simulink model "DoubleInvertedPendulum"  (R2015a)
settings: Solver=ode45  StartTime=0.0  StopTime=20  RelTol=1e-3
values from neighbouring files (symbols this model uses):
  A = [ ... (first row only)    [DoubleInvertedPendulum_config.m]
  B = [ ... (first row only)    [DoubleInvertedPendulum_config.m]
  g = 9.8    [DoubleInvertedPendulum_config.m]
  gain = lqr( A ,B, Q, R )    [DoubleInvertedPendulum_config.m]
  J1 = 1.0    (= 1)    [DoubleInvertedPendulum_config.m]
  J2 = 1.0    (= 1)    [DoubleInvertedPendulum_config.m]
  l1 = 2.0    (= 2)    [DoubleInvertedPendulum_config.m]
  l2 = 1.0    (= 1)    [DoubleInvertedPendulum_config.m]
  lg1 = 1.2    [DoubleInvertedPendulum_config.m]
  lg2 = 0.5    [DoubleInvertedPendulum_config.m]
  m0 = 5.0    (= 5)    [DoubleInvertedPendulum_config.m]
  m1 = 1.0    (= 1)    [DoubleInvertedPendulum_config.m]
  m2 = 1.0    (= 1)    [DoubleInvertedPendulum_config.m]
settings Model: Creator=hamada  LastModifiedBy=hamada

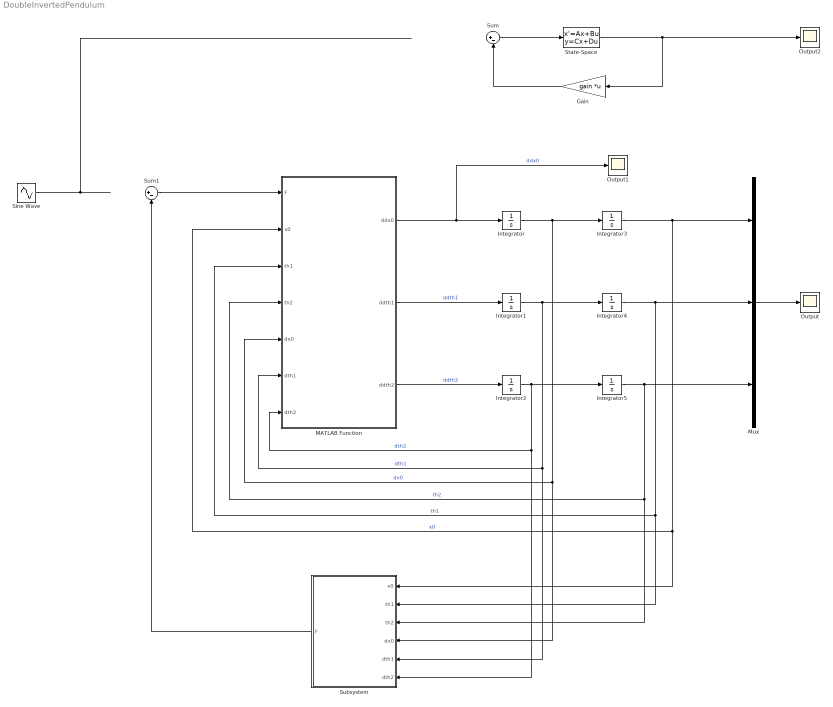
== system DoubleInvertedPendulum ==
  Gain : Gain  Gain=gain  Multiplication=Matrix(K*u)
  Integrator{,1..3} (4 alike) : Integrator
  Integrator4 : Integrator  InitialCondition=5*pi/180
  Integrator5 : Integrator  InitialCondition=5*pi/180
  MATLAB Function : MATLAB Function  TreatAsAtomicUnit=on
  Mux : Mux  Inputs=3
  Output : Scope
      settings: SaveName=Output  SampleInput=on  SampleTime=0.1
  Output1 : Scope
      settings: SaveName=Output1  SampleInput=on  SampleTime=0.1
  Output2 : Scope
      settings: SaveName=Output2  SampleInput=on  SampleTime=0.1
  Sine Wave : Sin  Amplitude=10  Frequency=1*2*pi  SampleTime=0
  State-Space : StateSpace  A=A  B=B  C=eye(6)  D=zeros(6,1)  X0=[0;5*pi/180;0;0;0;0]
  Subsystem : Subsystem
  Sum : Sum  Inputs=|+-
  Sum1 : Sum  Inputs=|+-
  wires:
  MATLAB Function/1(ddx0) -> Output1/1, Integrator/1  "ddx0"
  MATLAB Function/2(ddth1) -> Integrator1/1  "ddth1"
  MATLAB Function/3(ddth2) -> Integrator2/1  "ddth2"
  Integrator/1 -> Subsystem/4(dx0), MATLAB Function/5(dx0), Integrator3/1  "dx0"
  Integrator1/1 -> Subsystem/5(dth1), MATLAB Function/6(dth1), Integrator4/1  "dth1"
  Integrator2/1 -> Subsystem/6(dth2), MATLAB Function/7(dth2), Integrator5/1  "dth2"
  Integrator3/1 -> Mux/1, MATLAB Function/2(x0), Subsystem/1(x0)  "x0"
  Integrator4/1 -> Mux/2, Subsystem/2(th1), MATLAB Function/3(th1)  "th1"
  Integrator5/1 -> Subsystem/3(th2), MATLAB Function/4(th2), Mux/3  "th2"
  Sine Wave/1 -> ?
  Mux/1 -> Output/1
  State-Space/1 -> Output2/1, Gain/1
  Sum/1 -> State-Space/1
  Gain/1 -> Sum/2
  Sum1/1 -> MATLAB Function/1(F)
  Subsystem/1(F) -> Sum1/2

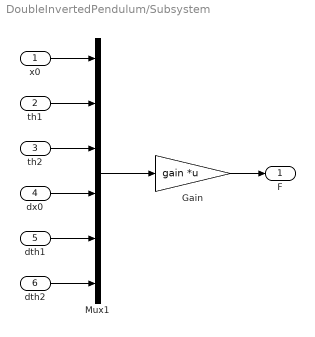
== system DoubleInvertedPendulum/Subsystem ==
  x0 : Inport
  th1 : Inport  Port=2
  th2 : Inport  Port=3
  dx0 : Inport  Port=4
  dth1 : Inport  Port=5
  dth2 : Inport  Port=6
  Gain : Gain  Gain=gain  Multiplication=Matrix(K*u)
  Mux1 : Mux  Inputs=6
  F : Outport
  wires:
  Mux1/1 -> Gain/1
  dth2/1 -> Mux1/6
  dx0/1 -> Mux1/4
  th1/1 -> Mux1/2
  dth1/1 -> Mux1/5
  x0/1 -> Mux1/1
  th2/1 -> Mux1/3
  Gain/1 -> F/1

== matlab function DoubleInvertedPendulum/MATLAB Function ==
  data: F input double size=1; x0 input double size=1; ddx0 output double size=1; ddth1 output double size=1; ddth2 output double size=1; th1 input double size=1; th2 input double size=1; dx0 input double size=1; dth1 input double size=1; dth2 input double size=1; lg1 parameter double size=1; l1 parameter double size=1; lg2 parameter double size=1; l2 parameter double size=1; m0 parameter double size=1; m1 parameter double size=1; m2 parameter double size=1; J1 parameter double size=1; J2 parameter double size=1; g parameter double size=1
function [ ddx0, ddth1, ddth2 ] = fcn( F, x0, th1, th2, dx0, dth1, dth2, lg1, l1, lg2, l2, m0, m1, m2, J1, J2, g )
    %#codegen
    ddx0 = (((g*l1^2*lg2^2*m2^3+(g*lg1^2*lg2^2*m1+J1*g*lg2^2)*m2^2)*cos(th2+th1)+(l1^2*lg2^3*m2^3*(cos(th2)^2-1)+(-lg1^2*lg2^3*m1-J1*lg2^3-J2*l1^2*lg2)*m2^2+(-J2*lg1^2*lg2*m1-J1*J2*lg2)*m2)*(dth2)^2+(dth1)*(l1^2*lg2^3*m2^3*(2*cos(th2)^2-2)+(-2*lg1^2*lg2^3*m1-2*J1*lg2^3-2*J2*l1^2*lg2)*m2^2+(-2*J2*lg1^2*lg2*m1-2*J1*J2*lg2)*m2)*(dth2)+(dth1)^2*(l1^2*lg2^3*m2^3*(cos(th2)^2-1)+(-lg1^2*lg2^3*m1-J1*lg2^3-J2*l1^2*lg2)*m2^2+(-J2*lg1^2*lg2*m1-J1*J2*lg2)*m2)+cos(th1)*(-g*l1^2*lg2^2*m2^3*cos(th2)-g*l1*lg1*lg2^2*m1*m2^2*cos(th2)))*sin(th2+th1)+(-l1^2*lg2^3*m2^3*cos(th2)*sin(th2)*(dth2)^2-2*l1^2*lg2^3*m2^3*(dth1)*cos(th2)*sin(th2)*(dth2)+(dth1)^2*(m2^3*(-l1^2*lg2^3*cos(th2)*sin(th2)-l1^3*lg2^2*sin(th2))+m2^2*(-l1*lg1^2*lg2^2*m1*sin(th2)-J1*l1*lg2^2*sin(th2)))+sin(th1)*(-g*l1^2*lg2^2*m2^3*cos(th2)-g*l1*lg1*lg2^2*m1*m2^2*cos(th2)))*cos(th2+th1)+cos(th1)*(m2^2*(l1*lg1*lg2^3*m1*sin(th2)+J2*l1^2*lg2*sin(th2))+l1^2*lg2^3*m2^3*sin(th2)+J2*l1*lg1*lg2*m1*m2*sin(th2))*(dth2)^2+cos(th1)*(dth1)*(m2^2*(2*l1*lg1*lg2^3*m1*sin(th2)+2*J2*l1^2*lg2*sin(th2))+2*l1^2*lg2^3*m2^3*sin(th2)+2*J2*l1*lg1*lg2*m1*m2*sin(th2))*(dth2)+(dth1)^2*(cos(th1)*(m2^2*(m1*(l1^2*lg1*lg2^2*cos(th2)*sin(th2)+l1*lg1*lg2^3*sin(th2))+J2*l1^2*lg2*sin(th2))+m2^3*(l1^3*lg2^2*cos(th2)*sin(th2)+l1^2*lg2^3*sin(th2))+J2*l1*lg1*lg2*m1*m2*sin(th2))+sin(th1)*(l1^3*lg2^2*m2^3*(cos(th2)^2-1)+m2^2*(lg2^2*m1*(l1^2*lg1*(cos(th2)^2-1)-l1*lg1^2)-J1*l1*lg2^2-J2*l1^3)+(-lg1^3*lg2^2*m1^2+(-J1*lg1*lg2^2-J2*l1*lg1^2-J2*l1^2*lg1)*m1-J1*J2*l1)*m2-J2*lg1^3*m1^2-J1*J2*lg1*m1))+F*l1^2*lg2^2*m2^2*(cos(th2)^2-1)+(g*l1^2*lg2^2*m2^3+(2*g*l1*lg1*lg2^2*m1+J2*g*l1^2)*m2^2+(g*lg1^2*lg2^2*m1^2+2*J2*g*l1*lg1*m1)*m2+J2*g*lg1^2*m1^2)*cos(th1)*sin(th1)+(-F*lg1^2*lg2^2*m1-F*J1*lg2^2-F*J2*l1^2)*m2-F*J2*lg1^2*m1-F*J1*J2)/((l1^2*lg2^2*m2^3+(lg1^2*lg2^2*m1+J1*lg2^2)*m2^2)*cos(th2+th1)^2+cos(th1)*(-2*l1^2*lg2^2*m2^3*cos(th2)-2*l1*lg1*lg2^2*m1*m2^2*cos(th2))*cos(th2+th1)+l1^2*lg2^2*m2^3*(cos(th2)^2-1)+m2^2*(l1^2*lg2^2*m0*(cos(th2)^2-1)+lg2^2*m1*(l1^2*(cos(th2)^2-1)-lg1^2)-J1*lg2^2-J2*l1^2)+(l1^2*lg2^2*m2^3+(2*l1*lg1*lg2^2*m1+J2*l1^2)*m2^2+(lg1^2*lg2^2*m1^2+2*J2*l1*lg1*m1)*m2+J2*lg1^2*m1^2)*cos(th1)^2+(-lg1^2*lg2^2*m1^2+(-lg1^2*lg2^2*m0-J1*lg2^2-J2*lg1^2-J2*l1^2)*m1+(-J1*lg2^2-J2*l1^2)*m0-J1*J2)*m2-J2*lg1^2*m1^2+(-J2*lg1^2*m0-J1*J2)*m1-J1*J2*m0);
    ddth1 = -(((l1*lg2^3*m2^3*cos(th2)*(dth2)^2+2*l1*lg2^3*m2^3*(dth1)*cos(th2)*(dth2)+l1*lg2^3*m2^3*(dth1)^2*cos(th2)+(g*l1*lg2^2*m2^3+g*lg1*lg2^2*m1*m2^2)*cos(th1))*cos(th2+th1)+(-l1*lg2^3*m2^3+(-lg1*lg2^3*m1-J2*l1*lg2)*m2^2-J2*lg1*lg2*m1*m2)*cos(th1)*(dth2)^2+(-2*l1*lg2^3*m2^3+(-2*lg1*lg2^3*m1-2*J2*l1*lg2)*m2^2-2*J2*lg1*lg2*m1*m2)*cos(th1)*(dth1)*(dth2)+m2^2*(-g*l1*lg2^2*m1*cos(th2)-g*l1*lg2^2*m0*cos(th2))-g*l1*lg2^2*m2^3*cos(th2)+(-l1*lg2^3*m2^3+(-lg1*lg2^3*m1-J2*l1*lg2)*m2^2-J2*lg1*lg2*m1*m2)*cos(th1)*(dth1)^2)*sin(th2+th1)+(-l1*lg2^3*m2^3*sin(th2)*(dth2)^2-2*l1*lg2^3*m2^3*(dth1)*sin(th2)*(dth2)-l1*lg2^3*m2^3*(dth1)^2*sin(th2)+(-g*l1*lg2^2*m2^3-g*lg1*lg2^2*m1*m2^2)*sin(th1))*cos(th2+th1)^2+((dth1)^2*(cos(th1)*(-l1^2*lg2^2*m2^3*sin(th2)-l1*lg1*lg2^2*m1*m2^2*sin(th2))+sin(th1)*(l1^2*lg2^2*m2^3*cos(th2)+l1*lg1*lg2^2*m1*m2^2*cos(th2)))+F*l1*lg2^2*m2^2*cos(th2))*cos(th2+th1)+(m2^2*(l1*lg2^3*m1*sin(th2)+l1*lg2^3*m0*sin(th2)+J2*l1*lg2*sin(th2))+m2*(J2*l1*lg2*m1*sin(th2)+J2*l1*lg2*m0*sin(th2))+l1*lg2^3*m2^3*sin(th2))*(dth2)^2+(dth1)*(m2^2*(2*l1*lg2^3*m1*sin(th2)+2*l1*lg2^3*m0*sin(th2)+2*J2*l1*lg2*sin(th2))+m2*(2*J2*l1*lg2*m1*sin(th2)+2*J2*l1*lg2*m0*sin(th2))+2*l1*lg2^3*m2^3*sin(th2))*(dth2)+(dth1)^2*(m2^2*(m1*(l1^2*lg2^2*cos(th2)*sin(th2)+l1*lg2^3*sin(th2))+m0*(l1^2*lg2^2*cos(th2)*sin(th2)+l1*lg2^3*sin(th2))+J2*l1*lg2*sin(th2))+m2^3*(l1^2*lg2^2*cos(th2)*sin(th2)+l1*lg2^3*sin(th2))+m2*(J2*l1*lg2*m1*sin(th2)+J2*l1*lg2*m0*sin(th2))+(-l1^2*lg2^2*m2^3+(-2*l1*lg1*lg2^2*m1-J2*l1^2)*m2^2+(-lg1^2*lg2^2*m1^2-2*J2*l1*lg1*m1)*m2-J2*lg1^2*m1^2)*cos(th1)*sin(th1))+(g*l1*lg2^2*m2^3+((g*lg1+g*l1)*lg2^2*m1+g*l1*lg2^2*m0+J2*g*l1)*m2^2+(g*lg1*lg2^2*m1^2+(g*lg1*lg2^2*m0+J2*g*lg1+J2*g*l1)*m1+J2*g*l1*m0)*m2+J2*g*lg1*m1^2+J2*g*lg1*m0*m1)*sin(th1)+(-F*l1*lg2^2*m2^2+(-F*lg1*lg2^2*m1-F*J2*l1)*m2-F*J2*lg1*m1)*cos(th1))/((l1^2*lg2^2*m2^3+(lg1^2*lg2^2*m1+J1*lg2^2)*m2^2)*cos(th2+th1)^2+cos(th1)*(-2*l1^2*lg2^2*m2^3*cos(th2)-2*l1*lg1*lg2^2*m1*m2^2*cos(th2))*cos(th2+th1)+l1^2*lg2^2*m2^3*(cos(th2)^2-1)+m2^2*(l1^2*lg2^2*m0*(cos(th2)^2-1)+lg2^2*m1*(l1^2*(cos(th2)^2-1)-lg1^2)-J1*lg2^2-J2*l1^2)+(l1^2*lg2^2*m2^3+(2*l1*lg1*lg2^2*m1+J2*l1^2)*m2^2+(lg1^2*lg2^2*m1^2+2*J2*l1*lg1*m1)*m2+J2*lg1^2*m1^2)*cos(th1)^2+(-lg1^2*lg2^2*m1^2+(-lg1^2*lg2^2*m0-J1*lg2^2-J2*lg1^2-J2*l1^2)*m1+(-J1*lg2^2-J2*l1^2)*m0-J1*J2)*m2-J2*lg1^2*m1^2+(-J2*lg1^2*m0-J1*J2)*m1-J1*J2*m0);
    ddth2 = ((((m2^3*(l1*lg2^3*cos(th2)+l1^2*lg2^2)+(lg1^2*lg2^2*m1+J1*lg2^2)*m2^2)*(dth2)^2+(dth1)*(m2^3*(2*l1*lg2^3*cos(th2)+2*l1^2*lg2^2)+(2*lg1^2*lg2^2*m1+2*J1*lg2^2)*m2^2)*(dth2)+(dth1)^2*(m2^3*(l1*lg2^3*cos(th2)+l1^2*lg2^2)+(lg1^2*lg2^2*m1+J1*lg2^2)*m2^2)+(g*l1*lg2^2*m2^3+g*lg1*lg2^2*m1*m2^2)*cos(th1))*cos(th2+th1)+cos(th1)*(m2^2*(m1*(-l1*lg1*lg2^2*cos(th2)-lg1*lg2^3)-J2*l1*lg2)+m2^3*(-l1^2*lg2^2*cos(th2)-l1*lg2^3)-J2*lg1*lg2*m1*m2)*(dth2)^2+cos(th1)*(dth1)*(m2^2*(m1*(-2*l1*lg1*lg2^2*cos(th2)-2*lg1*lg2^3)-2*J2*l1*lg2)+m2^3*(-2*l1^2*lg2^2*cos(th2)-2*l1*lg2^3)-2*J2*lg1*lg2*m1*m2)*(dth2)+cos(th1)*(dth1)^2*(m2^2*(m1*(-l1*lg1*lg2^2*cos(th2)-lg1*lg2^3)-J2*l1*lg2)+m2^3*(-l1^2*lg2^2*cos(th2)-l1*lg2^3)-J2*lg1*lg2*m1*m2)+m2^2*(m1*((-g*lg1^2-g*l1^2)*lg2-g*l1*lg2^2*cos(th2))+m0*(-g*l1*lg2^2*cos(th2)-g*l1^2*lg2)-J1*g*lg2)+m2^3*(-g*l1*lg2^2*cos(th2)-g*l1^2*lg2)+(g*l1^2*lg2*m2^3+2*g*l1*lg1*lg2*m1*m2^2+g*lg1^2*lg2*m1^2*m2)*cos(th1)^2+(-g*lg1^2*lg2*m1^2+(-g*lg1^2*lg2*m0-J1*g*lg2)*m1-J1*g*lg2*m0)*m2)*sin(th2+th1)+(-l1*lg2^3*m2^3*sin(th2)*(dth2)^2-2*l1*lg2^3*m2^3*(dth1)*sin(th2)*(dth2)-l1*lg2^3*m2^3*(dth1)^2*sin(th2)+(-g*l1*lg2^2*m2^3-g*lg1*lg2^2*m1*m2^2)*sin(th1))*cos(th2+th1)^2+(cos(th1)*(-l1^2*lg2^2*m2^3*sin(th2)-l1*lg1*lg2^2*m1*m2^2*sin(th2))*(dth2)^2+cos(th1)*(dth1)*(-2*l1^2*lg2^2*m2^3*sin(th2)-2*l1*lg1*lg2^2*m1*m2^2*sin(th2))*(dth2)+(dth1)^2*(cos(th1)*(-2*l1^2*lg2^2*m2^3*sin(th2)-2*l1*lg1*lg2^2*m1*m2^2*sin(th2))+sin(th1)*(m2^2*(m1*(l1*lg1*lg2^2*cos(th2)+(l1*lg1^2+l1^2*lg1)*lg2)+J1*l1*lg2)+m2^3*(l1^2*lg2^2*cos(th2)+l1^3*lg2)+(lg1^3*lg2*m1^2+J1*lg1*lg2*m1)*m2))+m2^2*(F*l1*lg2^2*cos(th2)+F*l1^2*lg2)+(-g*l1^2*lg2*m2^3-2*g*l1*lg1*lg2*m1*m2^2-g*lg1^2*lg2*m1^2*m2)*cos(th1)*sin(th1)+(F*lg1^2*lg2*m1+F*J1*lg2)*m2)*cos(th2+th1)+(m2^2*(m1*(l1^2*lg2^2*cos(th2)*sin(th2)+l1*lg2^3*sin(th2))+m0*(l1^2*lg2^2*cos(th2)*sin(th2)+l1*lg2^3*sin(th2))+J2*l1*lg2*sin(th2))+m2^3*(l1^2*lg2^2*cos(th2)*sin(th2)+l1*lg2^3*sin(th2))+m2*(J2*l1*lg2*m1*sin(th2)+J2*l1*lg2*m0*sin(th2)))*(dth2)^2+(dth1)*(m2^2*(m1*(2*l1^2*lg2^2*cos(th2)*sin(th2)+2*l1*lg2^3*sin(th2))+m0*(2*l1^2*lg2^2*cos(th2)*sin(th2)+2*l1*lg2^3*sin(th2))+2*J2*l1*lg2*sin(th2))+m2^3*(2*l1^2*lg2^2*cos(th2)*sin(th2)+2*l1*lg2^3*sin(th2))+m2*(2*J2*l1*lg2*m1*sin(th2)+2*J2*l1*lg2*m0*sin(th2)))*(dth2)+(dth1)^2*(m2^2*(m1*(lg2*(l1*lg1^2*sin(th2)+l1^3*sin(th2))+2*l1^2*lg2^2*cos(th2)*sin(th2)+l1*lg2^3*sin(th2))+m0*(2*l1^2*lg2^2*cos(th2)*sin(th2)+l1*lg2^3*sin(th2)+l1^3*lg2*sin(th2))+(J2+J1)*l1*lg2*sin(th2))+m2*(m1*(l1*lg1^2*lg2*m0*sin(th2)+(J2+J1)*l1*lg2*sin(th2))+l1*lg1^2*lg2*m1^2*sin(th2)+(J2+J1)*l1*lg2*m0*sin(th2))+m2^3*(2*l1^2*lg2^2*cos(th2)*sin(th2)+l1*lg2^3*sin(th2)+l1^3*lg2*sin(th2))+cos(th1)^2*(-l1^3*lg2*m2^3*sin(th2)-2*l1^2*lg1*lg2*m1*m2^2*sin(th2)-l1*lg1^2*lg2*m1^2*m2*sin(th2))+cos(th1)*sin(th1)*(m2*(m1^2*(-l1*lg1^2*lg2*cos(th2)-lg1^2*lg2^2)-2*J2*l1*lg1*m1)+m2^2*(m1*(-2*l1^2*lg1*lg2*cos(th2)-2*l1*lg1*lg2^2)-J2*l1^2)+m2^3*(-l1^3*lg2*cos(th2)-l1^2*lg2^2)-J2*lg1^2*m1^2))+sin(th1)*(m2*(m1*(m0*(g*l1*lg1*lg2*cos(th2)+g*lg1*lg2^2)+J2*g*lg1+J2*g*l1)+m1^2*(g*l1*lg1*lg2*cos(th2)+g*lg1*lg2^2)+J2*g*l1*m0)+m2^2*(m1*(lg2*(g*l1*lg1*cos(th2)+g*l1^2*cos(th2))+(g*lg1+g*l1)*lg2^2)+m0*(g*l1^2*lg2*cos(th2)+g*l1*lg2^2)+J2*g*l1)+m2^3*(g*l1^2*lg2*cos(th2)+g*l1*lg2^2)+J2*g*lg1*m1^2+J2*g*lg1*m0*m1)+cos(th1)*(m2*(m1*(-F*l1*lg1*lg2*cos(th2)-F*lg1*lg2^2)-F*J2*l1)+m2^2*(-F*l1^2*lg2*cos(th2)-F*l1*lg2^2)-F*J2*lg1*m1))/((l1^2*lg2^2*m2^3+(lg1^2*lg2^2*m1+J1*lg2^2)*m2^2)*cos(th2+th1)^2+cos(th1)*(-2*l1^2*lg2^2*m2^3*cos(th2)-2*l1*lg1*lg2^2*m1*m2^2*cos(th2))*cos(th2+th1)+l1^2*lg2^2*m2^3*(cos(th2)^2-1)+m2^2*(l1^2*lg2^2*m0*(cos(th2)^2-1)+lg2^2*m1*(l1^2*(cos(th2)^2-1)-lg1^2)-J1*lg2^2-J2*l1^2)+(l1^2*lg2^2*m2^3+(2*l1*lg1*lg2^2*m1+J2*l1^2)*m2^2+(lg1^2*lg2^2*m1^2+2*J2*l1*lg1*m1)*m2+J2*lg1^2*m1^2)*cos(th1)^2+(-lg1^2*lg2^2*m1^2+(-lg1^2*lg2^2*m0-J1*lg2^2-J2*lg1^2-J2*l1^2)*m1+(-J1*lg2^2-J2*l1^2)*m0-J1*J2)*m2-J2*lg1^2*m1^2+(-J2*lg1^2*m0-J1*J2)*m1-J1*J2*m0);
end
